simulink model "EvilSpagetty"  (R2020b)
settings: Solver=VariableStepAuto  StartTime=0.0  StopTime=3  RelTol=1e-3
(part 1 of 7)
settings Model: Creator=nels-  LastModifiedBy=nels-

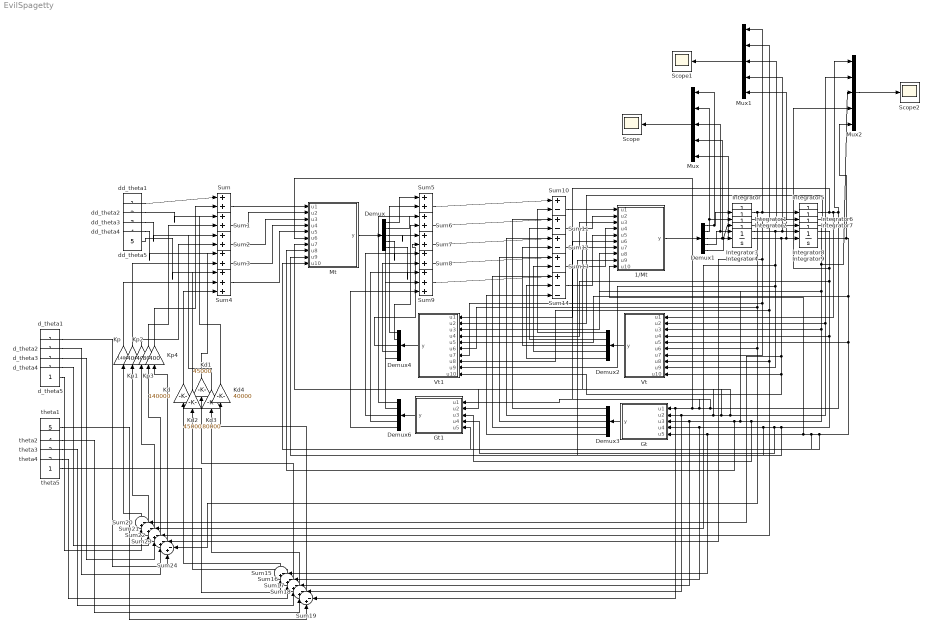
== system EvilSpagetty ==
  1/Mt : MATLAB Function  TreatAsAtomicUnit=on
  Demux{,1..4,6} (6 alike) : Demux  Outputs=5
  Gt : MATLAB Function  TreatAsAtomicUnit=on
  Gt1 : MATLAB Function  TreatAsAtomicUnit=on
  Integrator{,1..9} (10 alike) : Integrator
  Kd : Gain  Gain=140000
  Kd1 : Gain  Gain=45000
  Kd2 : Gain  Gain=45000
  Kd3 : Gain  Gain=80000
  Kd4 : Gain  Gain=40000
  Kp : Gain  Gain=1400
  Kp1 : Gain  Gain=400
  Kp2 : Gain  Gain=400
  Kp3 : Gain  Gain=800
  Kp4 : Gain  Gain=400
  Mt : MATLAB Function  TreatAsAtomicUnit=on
  Mux : Mux  Inputs=5
  Mux1 : Mux  Inputs=5
  Mux2 : Mux  Inputs=5
  Scope : Scope
  Scope1 : Scope
  Scope2 : Scope
  Sum{,1..9} (10 alike) : Sum  Inputs=|+++
  Sum{10..14} (5 alike) : Sum  Inputs=|+--
  Sum{15..24} (10 alike) : Sum  Inputs=|+-
  Vt : MATLAB Function  TreatAsAtomicUnit=on
  Vt1 : MATLAB Function  TreatAsAtomicUnit=on
  d_theta{1..5} (5 alike) : Constant
  dd_theta1 : Constant
  dd_theta2 : Constant  Value=2
  dd_theta3 : Constant  Value=3
  dd_theta4 : Constant  Value=4
  dd_theta5 : Constant  Value=5
  theta1 : Constant  Value=5
  theta2 : Constant  Value=4
  theta3 : Constant  Value=3
  theta4 : Constant  Value=2
  theta5 : Constant
  wires:
  dd_theta1/1 -> Sum/1
  dd_theta2/1 -> Sum1/1
  dd_theta3/1 -> Sum2/1
  dd_theta4/1 -> Sum3/1
  dd_theta5/1 -> Sum4/1
  Sum/1 -> Mt/1(u1)
  Sum1/1 -> Mt/2(u2)
  Sum2/1 -> Mt/3(u3)
  Sum3/1 -> Mt/4(u4)
  Sum4/1 -> Mt/5(u5)
  Mt/1(y) -> Demux/1
  Demux/1 -> Sum5/1
  Demux/2 -> Sum6/1
  Demux/3 -> Sum7/1
  Demux/4 -> Sum8/1
  Demux/5 -> Sum9/1
  Sum7/1 -> Sum12/1
  Sum8/1 -> Sum13/1
  Sum9/1 -> Sum14/1
  Sum10/1 -> 1/Mt/1(u1)
  Sum11/1 -> 1/Mt/2(u2)
  Sum12/1 -> 1/Mt/3(u3)
  Sum13/1 -> 1/Mt/4(u4)
  Sum14/1 -> 1/Mt/5(u5)
  1/Mt/1(y) -> Demux1/1
  Demux1/1 -> Mux/1, Integrator/1
  Demux1/2 -> Integrator1/1, Mux/2
  Demux1/3 -> Mux/4, Integrator2/1
  Integrator/1 -> Sum24/2, Vt/6(u6), Vt1/6(u6), Mux1/1, Integrator5/1
  Integrator2/1 -> Sum22/2, Vt/8(u8), Vt1/8(u8), Mux1/3, Integrator7/1
  Integrator3/1 -> Sum21/2, Vt1/9(u9), Vt/9(u9), Mux1/4, Integrator8/1
  Integrator6/1 -> Vt1/2(u2), Gt1/2(u2), 1/Mt/7(u7), Mt/7(u7), Sum18/2, Gt/2(u2), Vt/2(u2), Mux2/2
  Integrator8/1 -> Mux2/4, Vt1/4(u4), Mt/9(u9), Gt1/4(u4), 1/Mt/9(u9), Sum16/2, Gt/4(u4), Vt/4(u4)
  Integrator9/1 -> Mux2/5, Vt1/5(u5), Mt/10(u10), Gt1/5(u5), 1/Mt/10(u10), Sum15/2, Gt/5(u5), Vt/5(u5)
  Integrator4/1 -> Sum20/2, Vt1/10(u10), Vt/10(u10), Mux1/5, Integrator9/1
  Vt/1(y) -> Demux2/1
  Demux2/1 -> Sum10/2
  Demux2/3 -> Sum12/2
  Demux2/2 -> Sum11/2
  Demux2/4 -> Sum13/2
  Demux2/5 -> Sum14/2
  Gt/1(y) -> Demux3/1
  Demux3/1 -> Sum10/3
  Demux3/2 -> Sum11/3
  Demux3/3 -> Sum12/3
  Demux3/4 -> Sum13/3
  Demux3/5 -> Sum14/3
  Gt1/1(y) -> Demux6/1
  Vt1/1(y) -> Demux4/1
  Integrator5/1 -> Vt1/1(u1), Mux2/1, Gt1/1(u1), 1/Mt/6(u6), Mt/6(u6), Sum19/2, Gt/1(u1), Vt/1(u1)
  Integrator7/1 -> Mux2/3, Vt1/3(u3), Gt1/3(u3), 1/Mt/8(u8), Mt/8(u8), Sum17/2, Gt/3(u3), Vt/3(u3)
  Demux4/1 -> Sum5/2
  Demux4/2 -> Sum6/2
  Demux4/3 -> Sum7/2
  Demux4/4 -> Sum8/2
  Demux4/5 -> Sum9/2
  Demux6/1 -> Sum5/3
  Demux6/2 -> Sum6/3
  Demux6/3 -> Sum7/3
  Demux6/4 -> Sum8/3
  Demux6/5 -> Sum9/3
  theta1/1 -> Sum19/1
  theta2/1 -> Sum18/1
  Sum18/1 -> Kd3/1
  theta3/1 -> Sum17/1
  Sum17/1 -> Kd1/1
  theta4/1 -> Sum16/1
  Sum16/1 -> Kd2/1
  theta5/1 -> Sum15/1
  Sum15/1 -> Kd/1
  Sum19/1 -> Kd4/1
  Kd4/1 -> Sum/3
  Kd3/1 -> Sum1/3
  Kd1/1 -> Sum2/3
  Kd2/1 -> Sum3/3
  Kd/1 -> Sum4/3
  d_theta1/1 -> Sum24/1
  Integrator1/1 -> Sum23/2, Vt1/7(u7), Vt/7(u7), Mux1/2, Integrator6/1
  d_theta2/1 -> Sum23/1
  Sum24/1 -> Kp4/1
  Sum23/1 -> Kp3/1
  d_theta3/1 -> Sum22/1
  Sum22/1 -> Kp2/1
  d_theta4/1 -> Sum21/1
  Sum21/1 -> Kp1/1
  d_theta5/1 -> Sum20/1
  Sum20/1 -> Kp/1
  Kp4/1 -> Sum/2
  Kp3/1 -> Sum1/2
  Kp2/1 -> Sum2/2
  Kp1/1 -> Sum3/2
  Kp/1 -> Sum4/2
  Demux1/4 -> Mux/3, Integrator3/1
  Demux1/5 -> Mux/5, Integrator4/1
  Mux/1 -> Scope/1
  Mux1/1 -> Scope1/1
  Mux2/1 -> Scope2/1
  Sum5/1 -> Sum10/1
  Sum6/1 -> Sum11/1
